simulink model "Simulink_Model_2"  (R2025b)
settings: Solver=VariableStepAuto  StartTime=0.0  StopTime=10.0  RelTol=1e-3
values from neighbouring files (symbols this model uses):
  A = [0 1 0 0 ... (first row only)    [Matlab_Code.m]
  B = [0 0 ... (first row only)    [Matlab_Code.m]
  C = [1 0 0 0 ... (first row only)    [Matlab_Code.m]
  K = place(A,B_i,Pc)    [Matlab_Code.m]
  L = lT'    [Matlab_Code.m]
  Pend = Pend_parameters()    [Matlab_Code.m]
libraries: simulink_extras x2
settings Model: Creator=dburl  LastModifiedBy=dburl

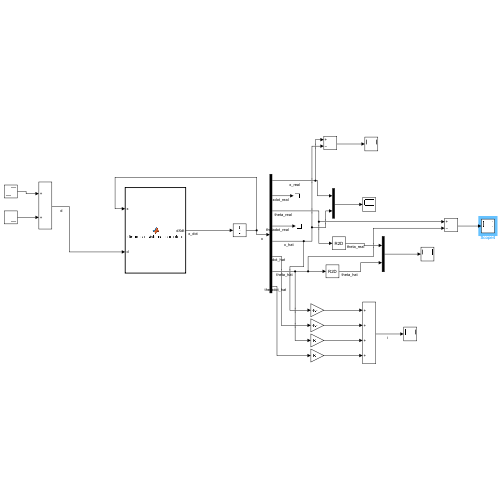
[thumbnail: Simulink's stored preview of the top-level diagram]
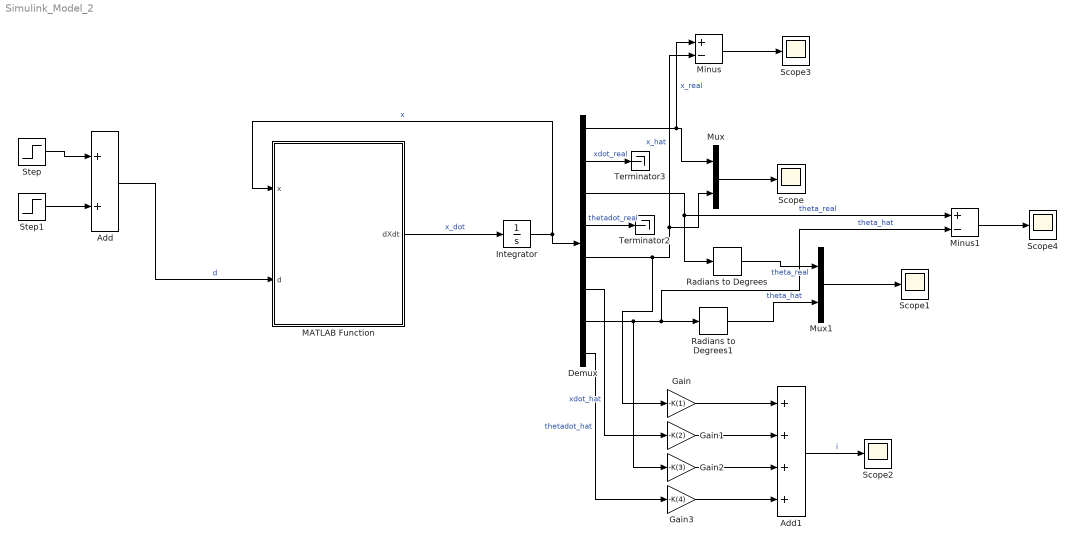
== system Simulink_Model_2 ==
  Add : Sum
  Add1 : Sum  Inputs=++++
  Demux : Demux  Outputs=8
  Gain : Gain  Gain=-K(1)
  Gain1 : Gain  Gain=-K(2)
  Gain2 : Gain  Gain=-K(3)
  Gain3 : Gain  Gain=-K(4)
  Integrator : Integrator  InitialCondition=[0;0;0;0;0;0;0;0]
  MATLAB Function : MATLAB Function  TreatAsAtomicUnit=on
  Minus : Sum  Inputs=+-
  Minus1 : Sum  Inputs=+-
  Mux : Mux  Inputs=2
  Mux1 : Mux  Inputs=2
  Radians to Degrees : simulink_extras/Transformations/Radians to Degrees
  Radians to Degrees1 : simulink_extras/Transformations/Radians to Degrees
  Scope{,1..4} (5 alike) : Scope
      Scope settings: ActiveDisplayYMinimum=-1  ActiveDisplayYMaximum=1
      Scope1 settings: ActiveDisplayYMinimum=-1  ActiveDisplayYMaximum=1
      Scope2 settings: ActiveDisplayYMinimum=-1  ActiveDisplayYMaximum=1  DataLoggingVariableName=ScopeData2
      Scope3 settings: ActiveDisplayYMinimum=-1  ActiveDisplayYMaximum=1  DataLoggingVariableName=ScopeData3
      Scope4 settings: ActiveDisplayYMinimum=-0.00064393164724422733  ActiveDisplayYMaximum=0.001971605442821333  DataLoggingVariableName=ScopeData4
  Step : Step  SampleTime=0
  Step1 : Step  Time=3  After=-1  SampleTime=0
  Terminator2 : Terminator
  Terminator3 : Terminator
  wires:
  Step/1 -> Add/1
  Step1/1 -> Add/2
  Add/1 -> MATLAB Function/2(d)  "d"
  MATLAB Function/1(dXdt) -> Integrator/1  "x_dot"
  Integrator/1 -> MATLAB Function/1(x), Demux/1  "x"
  Demux/1 -> Minus/1, Mux/1  "x_real"
  Demux/2 -> Terminator3/1  "xdot_real"
  Demux/3 -> Radians to Degrees/1, Minus1/1  "theta_real"
  Demux/4 -> Terminator2/1  "thetadot_real"
  Demux/5 -> Minus/2, Mux/2, Gain/1  "x_hat"
  Demux/6 -> Gain1/1  "xdot_hat"
  Demux/7 -> Minus1/2, Radians to Degrees1/1, Gain2/1  "theta_hat"
  Demux/8 -> Gain3/1  "thetadot_hat"
  Mux/1 -> Scope/1
  Mux1/1 -> Scope1/1
  Radians to Degrees1/1 -> Mux1/2  "theta_hat"
  Radians to Degrees/1 -> Mux1/1  "theta_real"
  Gain/1 -> Add1/1
  Gain1/1 -> Add1/2
  Gain2/1 -> Add1/3
  Gain3/1 -> Add1/4
  Add1/1 -> Scope2/1  "i"
  Minus/1 -> Scope3/1
  Minus1/1 -> Scope4/1

== matlab function Simulink_Model_2/MATLAB Function ==
  data: x input; Pend parameter; d input; dXdt output; A parameter; B parameter; C parameter; K parameter; L parameter
function dXdt = dinamica_sistema_completo(x,Pend,d,A, B, C, K, L)
    M = Pend.M;
    b = Pend.b;
    c = Pend.c;
    m = Pend.m;
    r = Pend.r;
    kt = Pend.kt;
    g = Pend.g;
    l = Pend.l;
    d0 = Pend.d0;
    am = kt/r;
    
    x_reale = x(1:4);   % [x; dx; theta; dtheta] veri
    x_stima = x(5:8);   % [x; dx; theta; dtheta] pensati dal microcontrollore
    
  
    % Il microcontrollore legge y dal mondo reale
    y = C * x_reale; 
    % --- IL CONTROLLORE (Motore) ---
    % Sceglie la corrente fidandosi SOLO della stima
    i = -K * x_stima;
    
    % --- IL DISTURBO (Task 2.2) ---
    % --- IL MONDO FISICO (Modello NON Lineare) ---
    % Estraiamo le variabili fisiche per comodità
    x1 = x_reale(1);
    x2 = x_reale(2);
    x3 = x_reale(3);
    x4 = x_reale(4);
    
    % QUI DEVI INSERIRE LE TUE FORMULE ESPLICITE DAL TASK 1.2
    % Nota: io scrivo "0" come segnaposto, ma tu devi usare le formule
    % che hai isolato per \ddot{x} e \ddot{\theta}
    accelerazione_carrello = (1/2*m*l*cos(x3)*((m*g*l/2)*sin(x3)-b*x4+d0*d*l^2/2*cos(x3))+1/3*m*l^2* ...
    (-1/2*m*l*(x4)^2*sin(x3)-c*x2+am*i-d0*l*d))/(1/3*m*(M+m)*l^2-1/4*m^2*l^2*cos(x3)^2); 
    accelerazione_angolo   = ((M+m)*(m*g*l/2*sin(x3)-b*x4+d0*d*l^2/2*cos(x3))+1/2*m*l*cos(x3)*...
    (-1/2*m*l*(x4)^2*sin(x3)-c*x2+am*i-d0*l*d))/(1/3*m*(M+m)*l^2-1/4*m^2*l^2*cos(x3)^2); 
    
    % Ricostruiamo il vettore delle derivate fisiche (4x1)
    xdot_reale = zeros(4,1);
    xdot_reale(1) = x_reale(2);                 % Velocità carrello
    xdot_reale(2) = accelerazione_carrello;     % Accelerazione carrello
    xdot_reale(3) = x_reale(4);                 % Velocità angolare
    xdot_reale(4) = accelerazione_angolo;       % Accelerazione angolare
    
    % --- IL MICROCONTROLLORE (Osservatore Lineare) ---
    % L'equazione di Luenberger aggiorna la stima internamente
    xdot_stima = A * x_stima + B(:,1) * i + L * (y - C * x_stima); %controllare colonne B
  
    % --- UNIONE DEL RISULTATO ---
    % Restituiamo a ode45 il super-vettore delle derivate (8x1)
    dXdt = [xdot_reale; xdot_stima];
